simulink model "malha"  (R2016a)
settings: Solver=VariableStepAuto  StartTime=0.0  StopTime=10.0  RelTol=1e-3
values from neighbouring files (symbols this model uses):
  croc = 0.001    [aeroservoelast.m]
  M_C = inv(M)*C    [aeroservoelast.m]
  M_FC = inv(M)*forca_no_cont    [aeroservoelast.m]
  M_FG = inv(M)*vento    [aeroservoelast.m]
  M_K = inv(M)*K    [aeroservoelast.m]
settings Model: Creator=Geraldo  LastModifiedBy=Geraldo

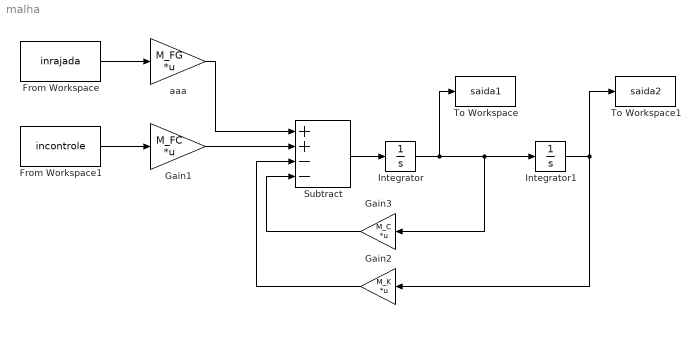
== system malha ==
  From Workspace : FromWorkspace  VariableName=inrajada  SampleTime=croc
  From Workspace1 : FromWorkspace  VariableName=incontrole  SampleTime=croc
  Gain1 : Gain  Gain=M_FC  Multiplication=Matrix(K*u) (u vector)
  Gain2 : Gain  Gain=M_K  Multiplication=Matrix(K*u)
  Gain3 : Gain  Gain=M_C  Multiplication=Matrix(K*u)
  Integrator : Integrator
  Integrator1 : Integrator
  Subtract : Sum  Inputs=++--
  To Workspace : ToWorkspace  VariableName=saida1  SampleTime=croc
  To Workspace1 : ToWorkspace  VariableName=saida2  SampleTime=croc
  aaa : Gain  Gain=M_FG  Multiplication=Matrix(K*u) (u vector)
  wires:
  From Workspace/1 -> aaa/1
  From Workspace1/1 -> Gain1/1
  aaa/1 -> Subtract/1
  Gain1/1 -> Subtract/2
  Gain2/1 -> Subtract/3
  Subtract/1 -> Integrator/1
  Integrator/1 -> To Workspace/1, Gain3/1, Integrator1/1
  Integrator1/1 -> To Workspace1/1, Gain2/1
  Gain3/1 -> Subtract/4
